simulink model "lcodi"  (Simulink 3.00)
settings: Solver=ode45  SolverMode=SingleTasking  StartTime=0.0  StopTime=20  MaxStep=.010  RelTol=1e-3  AbsTol=1e-3
undefined symbols (not defined in the file or in its folder): at, bt, ct, dt
settings Model: TimeSaveName=t  SaveOutput=off

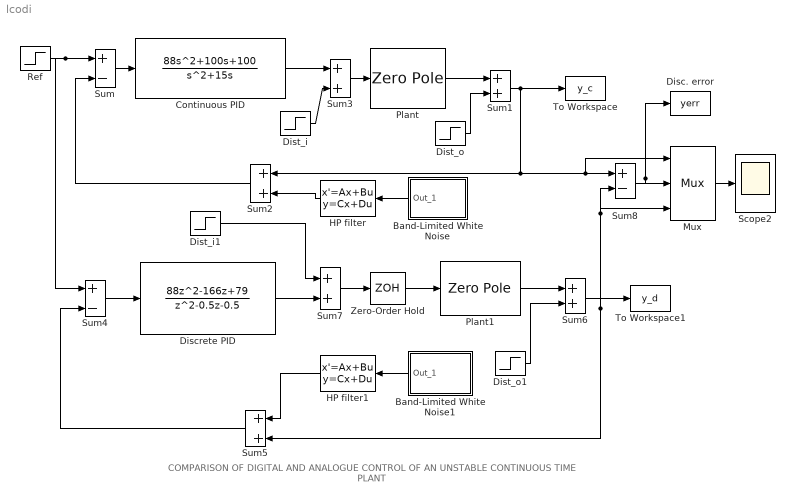
== system lcodi ==
  note: COMPARISON OF DIGITAL AND ANALOGUE CONTROL OF AN UNSTABLE CONTINUOUS TIME PLANT
  Band-Limited White Noise : Subsystem  Orientation=left  mask(Continuous White Noise.){@1=[0], @2=0.1, @3=[23341]}
      mask prompts: @1 "Noise Power:"; @2 "Sample Time:"; @3 "Seed"
      mask help:
      | White noise for continuous (s-domain) systems.
      | Band-limited using zero-order-hold.
      mask init:
      | Cov = @1; Ts = @2; seed = @3; r = rand(1,12); r2 = [r(1),r;r,r(12)]; t =[1:13;1:13];
      mask Help: Implemented using white noise into Zero-Order Hold block. The seed and power can be vectors of the same length to produce a vector of white noise sources. For faster simulation, set sample time to the highest value possible but in accordance with the fastest dynamics of system.
      mask Display: plot(t(:),r2(:))
  Band-Limited White Noise1 : Subsystem  Orientation=left  mask(Continuous White Noise.){@1=[0], @2=0.1, @3=[23341]}
      mask prompts: @1 "Noise Power:"; @2 "Sample Time:"; @3 "Seed"
      mask help:
      | White noise for continuous (s-domain) systems.
      | Band-limited using zero-order-hold.
      mask init:
      | Cov = @1; Ts = @2; seed = @3; r = rand(1,12); r2 = [r(1),r;r,r(12)]; t =[1:13;1:13];
      mask Help: Implemented using white noise into Zero-Order Hold block. The seed and power can be vectors of the same length to produce a vector of white noise sources. For faster simulation, set sample time to the highest value possible but in accordance with the fastest dynamics of system.
      mask Display: plot(t(:),r2(:))
  Continuous PID : TransferFcn  Numerator=[88 100 100]  Denominator=[1 15 0]
  Disc. error : ToWorkspace  VariableName=yerr  SampleTime=0  SaveFormat=Matrix
      settings: Buffer=10000
  Discrete PID : DiscreteTransferFcn  Numerator="[88  -166   79]"  Denominator="[1 -0.5  -0.5]"  SampleTime=0.1
  Dist_i : Step  Time=10  Before=0  After=1  SampleTime=0
  Dist_i1 : Step  Time=10  Before=0  After=1  SampleTime=0
  Dist_o : Step  Time=1  Before=0  After=0  SampleTime=0
  Dist_o1 : Step  Time=1  Before=0  After=0  SampleTime=0
  HP filter : StateSpace  Orientation=left  A=at  B=bt  C=ct  D=dt  X0=0  mask(buttap,lp2hp){@1=5, @2=4}
      mask prompts: @1 "Cutoff frequency (rad/sec):"; @2 "Order"
      mask help:
      | Analog Butterworth high pass filter.
      |
      | (Requires Signal Processing Toolbox)
      mask init:
      | [at,bt,ct,dt,w,mag]=filtm('buttap','lp2hp',@1,[],20,@2);
      mask Help: Butterworth high pass filter using MATLAB's butter and lp2hp commands.
      mask Display: plot(w,mag)
  HP filter1 : StateSpace  Orientation=left  A=at  B=bt  C=ct  D=dt  X0=0  mask(buttap,lp2hp){@1=5, @2=4}
      mask prompts: @1 "Cutoff frequency (rad/sec):"; @2 "Order"
      mask help:
      | Analog Butterworth high pass filter.
      |
      | (Requires Signal Processing Toolbox)
      mask init:
      | [at,bt,ct,dt,w,mag]=filtm('buttap','lp2hp',@1,[],20,@2);
      mask Help: Butterworth high pass filter using MATLAB's butter and lp2hp commands.
      mask Display: plot(w,mag)
  Mux : Mux  Inputs=3
      settings: DisplayOption=none
  Plant : ZeroPole  Zeros=[]  Poles=[1; 1]  Gain=[1]
  Plant1 : ZeroPole  Zeros=[]  Poles=[1; 1]  Gain=[1]
  Ref : Step  Time=1  Before=0  After=1  SampleTime=0
  Scope2 : Scope
      settings: TickLabels=on  TimeRange=20.000000  YMin=-0.4  YMax=0.4  SaveToWorkspace=off  SaveName=ScopeData  DataFormat=Matrix
  Sum : Sum  Inputs=+-  SaturateOnIntegerOverflow=on
  Sum{1,3,6..7} (4 alike) : Sum  Inputs=++  SaturateOnIntegerOverflow=on
  Sum2 : Sum  Orientation=left  Inputs=++  SaturateOnIntegerOverflow=on
  Sum4 : Sum  Inputs=+-  SaturateOnIntegerOverflow=on
  Sum5 : Sum  Orientation=left  Inputs=++  SaturateOnIntegerOverflow=on
  Sum8 : Sum  Inputs=+-  SaturateOnIntegerOverflow=on
  To Workspace : ToWorkspace  VariableName=y_c  SampleTime=0  SaveFormat=Matrix
      settings: Buffer=10000
  To Workspace1 : ToWorkspace  VariableName=y_d  SampleTime=0  SaveFormat=Matrix
      settings: Buffer=10000
  Zero-Order Hold : ZeroOrderHold  SampleTime=0.1
  wires:
  Sum/1 -> Continuous PID/1
  Sum3/1 -> Plant/1
  Mux/1 -> Scope2/1
  Sum2/1 -> Sum/2
  Sum1/1 -> To Workspace/1, Sum2/1, Sum8/1, Mux/1
  Sum8/1 -> Disc. error/1, Mux/2
  Sum4/1 -> Discrete PID/1
  Sum5/1 -> Sum4/2
  Band-Limited White Noise1/1(Out_1) -> HP filter1/1
  HP filter/1 -> Sum2/2
  Plant/1 -> Sum1/1
  Dist_o/1 -> Sum1/2
  Continuous PID/1 -> Sum3/1
  Dist_i/1 -> Sum3/2
  HP filter1/1 -> Sum5/1
  Sum6/1 -> Sum5/2, To Workspace1/1, Sum8/2, Mux/3
  Band-Limited White Noise/1(Out_1) -> HP filter/1
  Sum7/1 -> Zero-Order Hold/1
  Discrete PID/1 -> Sum7/2
  Dist_i1/1 -> Sum7/1
  Dist_o1/1 -> Sum6/2
  Zero-Order Hold/1 -> Plant1/1
  Plant1/1 -> Sum6/1
  Ref/1 -> Sum/1, Sum4/1

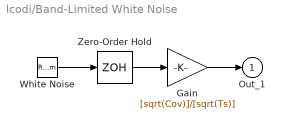
== system lcodi/Band-Limited White Noise ==
  Gain : Gain  Gain=[sqrt(Cov)]/[sqrt(Ts)]  SaturateOnIntegerOverflow=on
  White Noise : RandomNumber  Mean=0  Variance=1  Seed=seed  SampleTime=0
  Zero-Order Hold : ZeroOrderHold  SampleTime=Ts
  Out_1 : Outport  Port=1  InitialOutput=0
  wires:
  White Noise/1 -> Zero-Order Hold/1
  Gain/1 -> Out_1/1
  Zero-Order Hold/1 -> Gain/1

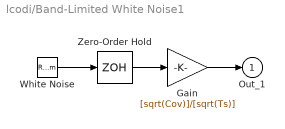
== system lcodi/Band-Limited White Noise1 ==
  Gain : Gain  Gain=[sqrt(Cov)]/[sqrt(Ts)]  SaturateOnIntegerOverflow=on
  White Noise : RandomNumber  Mean=0  Variance=1  Seed=seed  SampleTime=0
  Zero-Order Hold : ZeroOrderHold  SampleTime=Ts
  Out_1 : Outport  Port=1  InitialOutput=0
  wires:
  White Noise/1 -> Zero-Order Hold/1
  Gain/1 -> Out_1/1
  Zero-Order Hold/1 -> Gain/1
